simulink model "FM_Mod_Demod"  (R2024b)
settings: Solver=VariableStepAuto  StartTime=0.0  StopTime=10  RelTol=1e-3
libraries: dspfdesign x2, dspsrcs4 x2, commsynccomp2 x1
Description:
  | FM_Mod_Demod: This model simulate FM
  | Copyright (C) 2025  Mohammad Safa
  | GitHub Repository: https://github.com/mhr98/FM-Mod-Demod
  | 
  | This program is free software: you can redistribute it and/or modify
  | it under the terms of the GNU General Public License as published by
  | the Free Software Foundation, either version 3 of the License, or
  | (at your option) any later version.
  | 
  | This program is distributed in the hope that it will be useful,
  | but WITHOUT ANY WARRANTY; without even the implied warranty of
  | MERCHANTABILITY or FITNESS FOR A PARTICULAR PURPOSE.  See the
  | GNU General Public License for more details.
  | 
  | You should have received a copy of the GNU General Public License
  | along with this program.  If not, see <https://www.gnu.org/licenses/>.
settings Model: Creator=ASUS  LastModifiedBy=ASUS

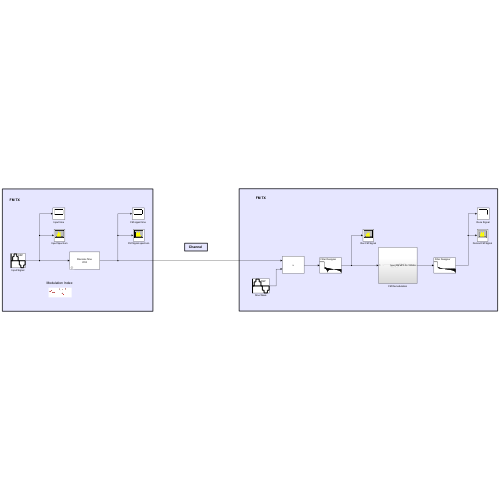
[thumbnail: Simulink's stored preview of the top-level diagram]
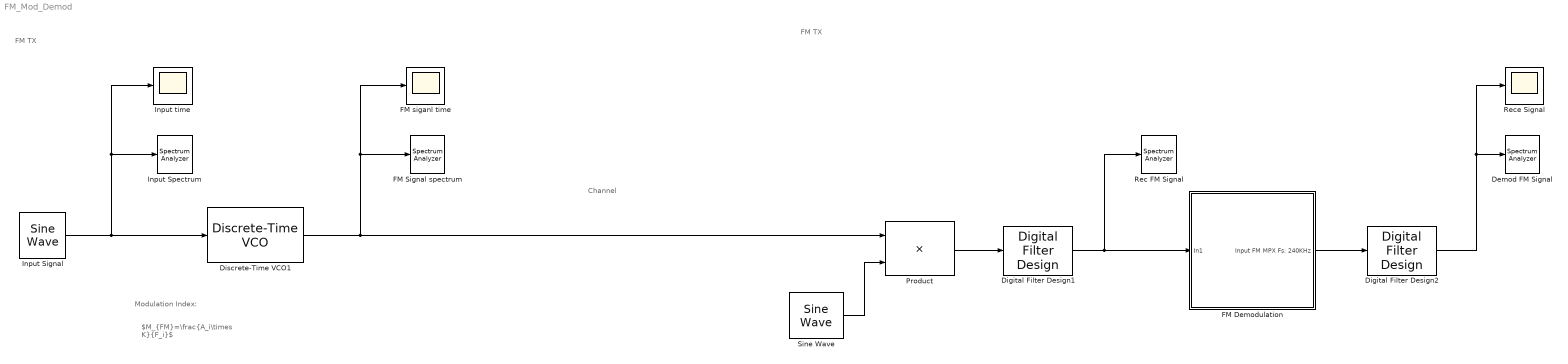
== system FM_Mod_Demod ==
  note: Channel
  note: FM TX
  note: FM TX
  note: Modulation Index:
  note: $M_{FM}=\frac{A_i\times K}{F_i}$
  Demod FM Signal : SpectrumAnalyzer  WindowPosition=[400.000000,294.000000,736.000000,277.000000,]  ScopeFrameLocation=window  AxesScaling=Manual  WindowInvariantSamplesPerUpdate=on  Span=48000  StartFrequency=-24000  StopFrequency=24000  YLimits=[-50 50]
  Digital Filter Design1 : dspfdesign/Digital Filter Design  mwdsp_browser_bugfix_var=off
  Digital Filter Design2 : dspfdesign/Digital Filter Design  mwdsp_browser_bugfix_var=off
  Discrete-Time VCO1 : commsynccomp2/Discrete-Time VCO  Ac=1  Fc=15e3  Kc=800  Ph=0  ts=1/48000
  FM Demodulation : Subsystem
  FM Signal spectrum : SpectrumAnalyzer  WindowPosition=[3.000000,298.000000,734.000000,254.000000,]  ScopeFrameLocation=window  AxesScaling=Manual  WindowInvariantSamplesPerUpdate=on  YLimits=[-50 50]
  FM siganl time : Scope
  Input Signal : dspsrcs4/Sine Wave  Amplitude=1  Frequency=400  Phase=0  SampleMode=Discrete  OutComplex=Real  CompMethod=Trigonometric fcn  TableSize=Speed  SampleTime=1/48e3  SamplesPerFrame=1  ResetState=Restart at time zero  OutputFrames=off  dataType=double  wordLen=16  udDataType=sfix(16)  fracBitsMode=Best precision  numFracBits=15  OutDataTypeStr=double  LastOutDataTypeStr=double
  Input Spectrum : SpectrumAnalyzer  WindowPosition=[405.000000,312.000000,727.000000,240.000000,]  ScopeFrameLocation=window  AxesScaling=Manual  WindowInvariantSamplesPerUpdate=on  Span=48000  StartFrequency=-24000  StopFrequency=24000  YLimits=[-50 50]
  Input time : Scope
  Product : Product
  Rec FM Signal : SpectrumAnalyzer  WindowPosition=[-35.000000,-25.000000,743.000000,271.000000,]  ScopeFrameLocation=window  AxesScaling=Manual  WindowInvariantSamplesPerUpdate=on  Span=48000  StartFrequency=-24000  StopFrequency=24000  YLimits=[-50 40]
  Rece Signal : Scope
  Sine Wave : dspsrcs4/Sine Wave  Amplitude=1  Frequency=15e3  Phase=0  SampleMode=Discrete  OutComplex=Complex  CompMethod=Trigonometric fcn  TableSize=Speed  SampleTime=1/48000  SamplesPerFrame=1  ResetState=Restart at time zero  OutputFrames=off  dataType=double  wordLen=16  udDataType=sfix(16)  fracBitsMode=Best precision  numFracBits=15  OutDataTypeStr=double  LastOutDataTypeStr=double
  wires:
  Input Signal/1 -> Discrete-Time VCO1/1, Input time/1, Input Spectrum/1
  FM Demodulation/1(Input FM MPX Fs: 240KHz) -> Digital Filter Design2/1
  Product/1 -> Digital Filter Design1/1
  Sine Wave/1 -> Product/2
  Digital Filter Design1/1 -> Rec FM Signal/1, FM Demodulation/1(In1)
  Digital Filter Design2/1 -> Rece Signal/1, Demod FM Signal/1
  Discrete-Time VCO1/1 -> Product/1, FM siganl time/1, FM Signal spectrum/1

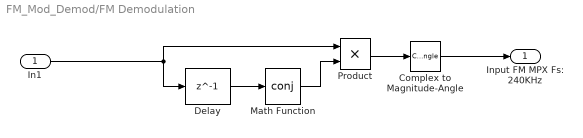
== system FM_Mod_Demod/FM Demodulation ==
  In1 : Inport
  Complex to Magnitude-Angle : ComplexToMagnitudeAngle  Output=Angle
  Delay : Delay  DelayLength=1  InputProcessing=Columns as channels (frame based)
  Math Function : Math  Operator=conj
  Product : Product
  Input FM MPX Fs: 240KHz : Outport
  wires:
  In1/1 -> Delay/1, Product/1
  Delay/1 -> Math Function/1
  Math Function/1 -> Product/2
  Complex to Magnitude-Angle/1 -> Input FM MPX Fs: 240KHz/1
  Product/1 -> Complex to Magnitude-Angle/1
